simulink subsystem "StudentTemplate_M2"  (R2025a)
settings: Solver=VariableStepAuto  StartTime=0.0  StopTime=10.0  RelTol=1e-3
libraries: simulink x5, eeGeneralControl x3, slpidlib x2
settings Model: Creator=JesseJabezArendse  LastModifiedBy=MTMTAD006

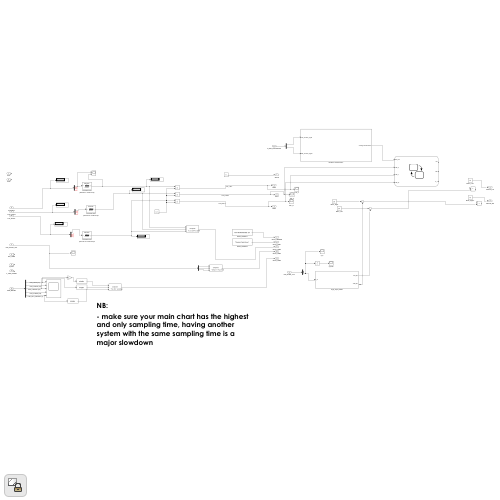
[thumbnail: Simulink's stored preview of the top-level diagram]
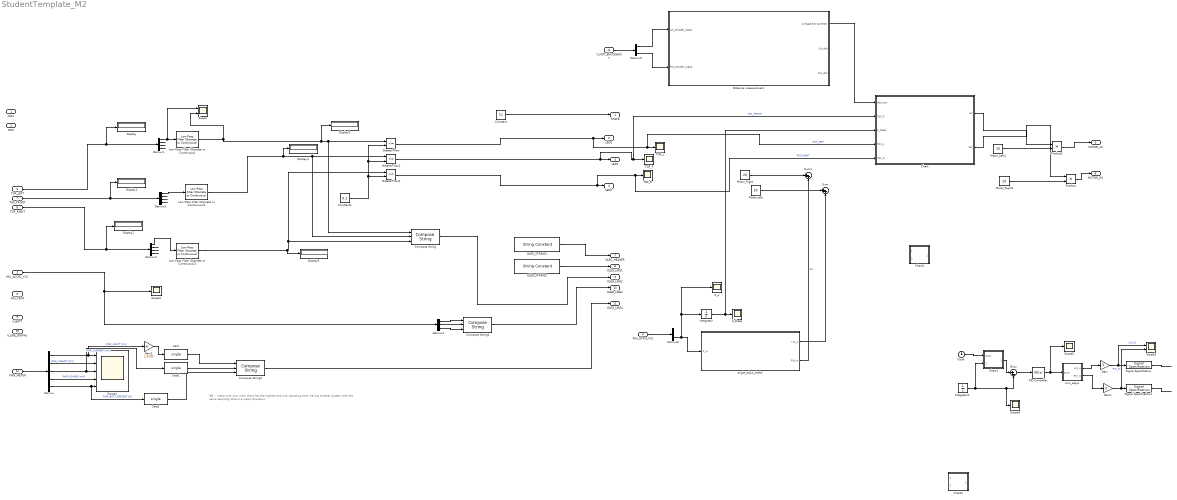
== system StudentTemplate_M2 ==
  note: NB:
      |
      | - make sure your main chart has the highest and only sampling time, having another system with the same sampling time is a major slowdown
  SW1 : Inport
  SW2 : Inport  Port=2
  IMU_ACCEL_XYZ : Inport  Port=3
  IMU_GYRO_XYZ : Inport  Port=4
  IMU_TEMP : Inport  Port=5
  TOF_LEFT : Inport  Port=6
  TOF_FRONT : Inport  Port=7
  TOF_RIGHT : Inport  Port=8
  V_BATT : Inport  Port=9
  V_LINE_DOWNs : Inport  Port=10
  V_MOT_ENCODERSs : Inport  Port=11
  PWR_METER : Inport  Port=12
  Cast : DataTypeConversion  OutDataTypeStr=single  SaturateOnIntegerOverflow=off  RndMeth=Floor
  Cast1 : DataTypeConversion  OutDataTypeStr=single  SaturateOnIntegerOverflow=off  RndMeth=Floor
  Cast2 : DataTypeConversion  OutDataTypeStr=single  SaturateOnIntegerOverflow=off  RndMeth=Floor
  Chart : Stateflow chart  TreatAsAtomicUnit=on
      settings: PortSchema="{\"entries\":[{\"content\":{\"sides\":[{\"content\":{\"connectorIds\":[\"In3\",\"In4\",\"In5\",\"In1\",\"In2\"]},\"type\":\"ConnectorPlacement.EquallySpacedRectSide\",\"uuid\":\"48a59af2-7c84-427a-8e2f-b10f2a044ed3\"},{\"content\":{\"connectorIds\":[\"Out1\",\"Out2\"],\"side\":\"RIGHT\"},\"type\":\"ConnectorPlacement.EquallySpacedRectSide\",\"uuid\":\"ddb5ed95-9874-42e8-8fee-75458ccb7c53\"},{\"content\":{\"side\":\"TOP\"},\"type\":\"ConnectorPlacement.EquallySpacedRectSide\",\"uuid\":\"d57417fe-864c-49b1-b704-1964fc5ecc42\"}]},\"type\":\"ConnectorPlacement.EquallySpacedConnector\",\"uuid\":\"f24c4a6d-faf6-462a-ab68-e289d44b6927\"}],\"packageUris\":[\"http://schema.mathworks.com/mf0/Connector/R2020b\"],\"version\":\"1.0\"}"
  Chart1 : Stateflow chart  TreatAsAtomicUnit=on
  Chart2 : Stateflow chart  TreatAsAtomicUnit=on
  Chart3 : Stateflow chart  TreatAsAtomicUnit=on
  Clock : Clock
  Compose String : ComposeString  Format="\"L%1.2f F%1.2f R%1.2f\""
  Compose String1 : ComposeString  Format="\"X%2.1f  Y%2.1f  Z%2.1f\""
  Compose String2 : ComposeString  Format="\"%1.2fV  %3.0fmA  %2.0f%%\""
  Constant : Constant  Value=11
  Constant1 : Constant  Value=0.1  SampleTime=-1
  "DIstance measurement " : Subsystem
  Demux : Demux  Outputs=5
  Demux1 : Demux
  Demux2 : Demux
  Demux3 : Demux
  Demux4 : Demux  Outputs=3
  Demux5 : Demux  Outputs=2
  Demux6 : Demux  Outputs=3
  Display{,1..5} (6 alike) : Display
  Error : Sum  Inputs=|+-
  Gain : Gain  Gain=5
  Gain1 : Gain  Gain=5
  Gain2 : Gain  Gain=1/1000
  GreaterThan : RelationalOperator  Operator=<=  OutDataTypeStr=boolean  RndMeth=Simplest  InputSameDT=off
  GreaterThan1 : RelationalOperator  Operator=<=  OutDataTypeStr=boolean  RndMeth=Simplest  InputSameDT=off
  GreaterThan2 : RelationalOperator  Operator=<=  OutDataTypeStr=boolean  RndMeth=Simplest  InputSameDT=off
  Integrator : Integrator
  Integrator1 : Integrator
  Low-Pass Filter (Discrete or Continuous) : eeGeneralControl/Low-Pass Filter (Discrete or Continuous)  K=1  T=0.1  B=inf  A=-inf  init_option=Inherited from block input  x0=0  Ts=-1
  Low-Pass Filter (Discrete or Continuous)1 : eeGeneralControl/Low-Pass Filter (Discrete or Continuous)  K=1  T=0.1  B=inf  A=-inf  init_option=Inherited from block input  x0=0  Ts=-1
  Low-Pass Filter (Discrete or Continuous)2 : eeGeneralControl/Low-Pass Filter (Discrete or Continuous)  K=1  T=0.1  B=inf  A=-inf  init_option=Inherited from block input  x0=0  Ts=-1
  Motor_Left : Constant  Value=20
  Motor_Left1 : Constant  Value=20
  Motor_Right : Constant  Value=20
  Motor_Right1 : Constant  Value=20
  OLED_STRING1 : StringConstant  String="\"UCT MICROMOUSE '25\""
  OLED_STRING2 : StringConstant  String="\"Simulink Data Demo\""
  PID Controller : slpidlib/PID Controller  Controller=PD  Form=Parallel  TimeDomain=Continuous-time  UseExternalTs=off  SampleTime=-1  IntegratorMethod=Forward Euler  FilterMethod=Forward Euler  ControllerParametersSource=internal  P=50  I=1  UseKiTs=off  D=1  UseExternalDerivativeSource=off  N=100  UseFilter=on  TunerSelectOption=Transfer Function Based (PID Tuner App)  InitialConditionSource=internal  InitialConditionForIntegrator=0  InitialConditionForFilter=0  DifferentiatorICPrevScaledInput=0  ExternalReset=none  TrackingMode=off  Kt=1  LimitOutput=off  SatLimitsSource=internal  UpperSaturationLimit=inf  LowerSaturationLimit=-inf  LinearizeAsGain=on  AntiWindupMode=none  Kb=1  LimitIntegrator=off  UpperIntegratorSaturationLimit=inf  LowerIntegratorSaturationLimit=-inf  POutMin=[]  POutMax=[]  IOutMin=[]  IOutMax=[]  DOutMin=[]  DOutMax=[]  NOutMin=[]  NOutMax=[]  SumOutMin=[]  SumOutMax=[]  SaturationOutMin=[]  SaturationOutMax=[]  PParamMin=[]  PParamMax=[]  IParamMin=[]  IParamMax=[]  DParamMin=[]  DParamMax=[]  NParamMin=[]  NParamMax=[]  KbParamMin=[]  KbParamMax=[]  KtParamMin=[]  KtParamMax=[]  KbOutMin=[]  KbOutMax=[]  KtOutMin=[]  KtOutMax=[]  IntegratorOutMin=[]  IntegratorOutMax=[]  FilterOutMin=[]  FilterOutMax=[]  SumI1OutMin=[]  SumI1OutMax=[]  SumI2OutMin=[]  SumI2OutMax=[]  SumI3OutMin=[]  SumI3OutMax=[]  SumI4OutMin=[]  SumI4OutMax=[]  SumDOutMin=[]  SumDOutMax=[]  DifferentiatorOutMin=[]  DifferentiatorOutMax=[]  FilterDiffOutCoefMin=[]  FilterDiffOutCoefMax=[]  ReciprocalOutMin=[]  ReciprocalOutMax=[]  SumDenOutMin=[]  SumDenOutMax=[]  SumNumOutMin=[]  SumNumOutMax=[]  DivideOutMin=[]  DivideOutMax=[]  UdiffTsProdOutMin=[]  UdiffTsProdOutMax=[]  NTsProdOutMin=[]  NTsProdOutMax=[]  UintegralTsProdOutMin=[]  UintegralTsProdOutMax=[]  UngainTsProdOutMin=[]  UngainTsProdOutMax=[]  ClampingZeroOutDataTypeStr=Inherit: Inherit via back propagation  ClampingZeroOutMin=[]  ClampingZeroOutMax=[]  FilterDenConstantOutDataTypeStr=Inherit: Inherit via back propagation  FilterDenConstantOutMin=[]  FilterDenConstantOutMax=[]  PCopyOutDataTypeStr=Inherit: Inherit via back propagation  PCopyOutMin=[]  PCopyOutMax=[]  NCopyOutDataTypeStr=Inherit: Inherit via back propagation  NCopyOutMin=[]  NCopyOutMax=[]  IntegratorContinuousStateAttributes=''  IntegratorStateMustResolveToSignalObject=off  IntegratorRTWStateStorageClass=Auto  FilterContinuousStateAttributes=''  FilterStateMustResolveToSignalObject=off  FilterRTWStateStorageClass=Auto  ParallelPVariant=InternalParameters  IdealPVariant=Disabled  IVariant=Disabled  DVariant=InternalParameters  IntegratorVariant=Disabled  SatVariant=Disabled  AWVariant=Disabled  PCopyVariant=Disabled  TRVariant=Disabled  FdbkBlocksVariant=Forward  IdealPFdbkVariant=Disabled  SatFdbkVariant=Disabled  DerivativeFilterVariant=ContFilter  NVariant=InternalParameters  NCopyVariant=Disabled  FilterICVariant=InternalICsFilter  IntegratorICVariant=Disabled  ExternalResetVariant=Disabled  TRSumVariant=Passthrough  SumFdbkVariant=Disabled  SumVariant=Sum_PD  TsampFilterVariant=InternalTs  TsampNgainVariant=Passthrough  TsampIntegralVariant=Disabled_SignalSpec  ExternalSaturationOutDataTypeStr=Inherit: Same as second input  DerivativeSourceVariant=ErrorSignal  PreIntVariant=InternalPreInt
  Product : Product
  Product1 : Product
  Scope : Scope  NumInputPorts=2
      settings: ActiveDisplayYMinimum=0.22759  ActiveDisplayYMaximum=0.52326
  Scope1 : Scope  NumInputPorts=5
      settings: ActiveDisplayYMinimum=-437.5  ActiveDisplayYMaximum=3937.5  DataLoggingVariableName=ScopeData2
  Scope2 : Scope
  Scope3 : Scope  NumInputPorts=2
      settings: ActiveDisplayYMinimum=-440.40684872460486  ActiveDisplayYMaximum=398.93122569343797  DataLoggingVariableName=ScopeData11
  Scope4 : Scope
      settings: ActiveDisplayYMinimum=-2.1976138852237335  ActiveDisplayYMaximum=0.12970641062525379  DataLoggingVariableName=ScopeData14
  Scope5 : Scope
      settings: ActiveDisplayYMinimum=-4.4488284675734473  ActiveDisplayYMaximum=3.9249085751009725  DataLoggingVariableName=ScopeData16
  Signal Specification : SignalSpecification  Dimensions=1
  Signal Specification1 : SignalSpecification  Dimensions=1
  Sum : Sum  Inputs=|++
  Sum1 : Sum  Inputs=|++
  TOF_F : Scope
      settings: ActiveDisplayYMinimum=-0.1769980412947128  ActiveDisplayYMaximum=0.90279895686963285  DataLoggingVariableName=ScopeData4
  TOF_L : Scope
      settings: ActiveDisplayYMinimum=-0.062899688908756052  ActiveDisplayYMaximum=0.13734742485444948  DataLoggingVariableName=ScopeData3
  TOF_R : Scope
      settings: ActiveDisplayYMinimum=0.84085955530656642  ActiveDisplayYMaximum=1.1222796398378163  DataLoggingVariableName=ScopeData5
  Z_theta : Scope
      settings: ActiveDisplayYMinimum=-2.70161604115423  ActiveDisplayYMaximum=4.8892356554264911  DataLoggingVariableName=ScopeData7
  Z_w : Scope
      settings: ActiveDisplayYMinimum=0.15654767663707053  ActiveDisplayYMaximum=0.20860795869615065  DataLoggingVariableName=ScopeData6
  angle_adjus_draft2 : Subsystem
  turn_adjus : Stateflow chart  TreatAsAtomicUnit=on
  STATE : Outport
  LED0 : Outport  Port=2
  LED1 : Outport  Port=3
  LED2 : Outport  Port=4
  MOTOR_LS : Outport  Port=5
  MOTOR_RS : Outport  Port=6
  OLED_HEADER : Outport  Port=7
  OLED_LINE1 : Outport  Port=8
  OLED_LINE2 : Outport  Port=9
  OLED_LINE3 : Outport  Port=10
  OLED_LINE4 : Outport  Port=11
  wires:
  TOF_FRONT/1 -> Demux3/1, Display1/1
  OLED_STRING2/1 -> OLED_LINE1/1
  Demux2/1 -> Low-Pass Filter (Discrete or Continuous)2/1
  Demux2/3 -> ?
  Demux2/2 -> ?
  Demux2/4 -> ?
  Compose String1/1 -> OLED_LINE3/1
  Low-Pass Filter (Discrete or Continuous)1/1 -> Compose String/2, GreaterThan1/1, Display4/1
  GreaterThan1/1 -> LED1/1, TOF_F/1, Chart/4(TOF_F)  "TOF_FRONT"
  Demux3/3 -> ?
  TOF_RIGHT/1 -> Demux2/1, Display2/1
  Demux3/4 -> ?
  Demux3/2 -> ?
  Demux1/2 -> ?
  Demux3/1 -> Low-Pass Filter (Discrete or Continuous)1/1
  OLED_STRING1/1 -> OLED_HEADER/1
  Demux1/1 -> Scope/1, Low-Pass Filter (Discrete or Continuous)/1
  Compose String/1 -> OLED_LINE2/1
  Constant1/1 -> GreaterThan2/2, GreaterThan1/2, GreaterThan/2
  Demux1/4 -> ?
  GreaterThan2/1 -> TOF_R/1, Chart/2(TOF_R), LED2/1  "TOF_RIGHT"
  TOF_LEFT/1 -> Demux1/1, Display/1
  GreaterThan/1 -> LED0/1, TOF_L/1, Chart/1(TOF_L)  "TOF_LEFT"
  Demux1/3 -> ?
  PWR_METER/1 -> Demux/1
  Demux/1 -> Scope1/1, Gain2/1  "PWR_VBATT [mV]"
  Demux/2 -> Scope1/2  "PWR_VSHUNT [mV]"
  Demux/3 -> Scope1/3, Cast1/1  "PWR_CURRENT [mA]"
  Demux/4 -> Scope1/4  "PWR_POWER [mW]"
  Demux/5 -> Scope1/5, Cast2/1  "PWR_BATT_PERCENT [%]"
  IMU_ACCEL_XYZ/1 -> Demux4/1, Scope2/1
  Demux4/1 -> Compose String1/1
  Demux4/2 -> Compose String1/2
  Demux4/3 -> Compose String1/3
  Compose String2/1 -> OLED_LINE4/1
  Gain2/1 -> Cast/1
  Cast/1 -> Compose String2/1
  Cast1/1 -> Compose String2/2
  Cast2/1 -> Compose String2/3
  Low-Pass Filter (Discrete or Continuous)2/1 -> Compose String/3, GreaterThan2/1, Display5/1
  Low-Pass Filter (Discrete or Continuous)/1 -> Scope/2, Compose String/1, GreaterThan/1, Display3/1
  Constant/1 -> STATE/1
  Motor_Right/1 -> Sum1/1
  V_MOT_ENCODERSs/1 -> Demux5/1
  Demux5/1 -> "DIstance measurement "/1(LW_encoder_signal)
  Demux5/2 -> "DIstance measurement "/2(RW_encoder_signal)
  IMU_GYRO_XYZ/1 -> Demux6/1
  Demux6/3 -> angle_adjus_draft2/1(Z_w), Integrator/1, Z_w/1
  Motor_Left/1 -> Sum/1
  angle_adjus_draft2/1(LW_w) -> Sum/2
  angle_adjus_draft2/2(RW_w) -> Sum1/2  "RW"
  Motor_Left1/1 -> Product1/2
  Motor_Right1/1 -> Product/2
  "DIstance measurement "/1("Average dist tarvelled ") -> Chart/3(dist_trav)
  Product1/1 -> MOTOR_LS/1
  Product/1 -> MOTOR_RS/1
  Integrator/1 -> Z_theta/1, Chart/5(Z_theta)
  Chart/2(RW) -> Product/1
  Chart/1(LW) -> Product1/1
  Clock/1 -> Chart1/1(clock)
  Error/1 -> PID Controller/1
  Signal Specification/1 -> ?
  turn_adjus/1(LW_w) -> Gain/1
  turn_adjus/2(RW_w) -> Gain1/1
  Gain1/1 -> Signal Specification1/1, Scope3/2  "RW_W"
  Integrator1/1 -> Error/2, Scope4/1, Chart1/2(Z_theta)
  Chart1/1(offset) -> Error/1
  Signal Specification1/1 -> ?
  PID Controller/1 -> turn_adjus/1(error), Scope5/1
  Gain/1 -> Signal Specification/1, Scope3/1  "LW_W"

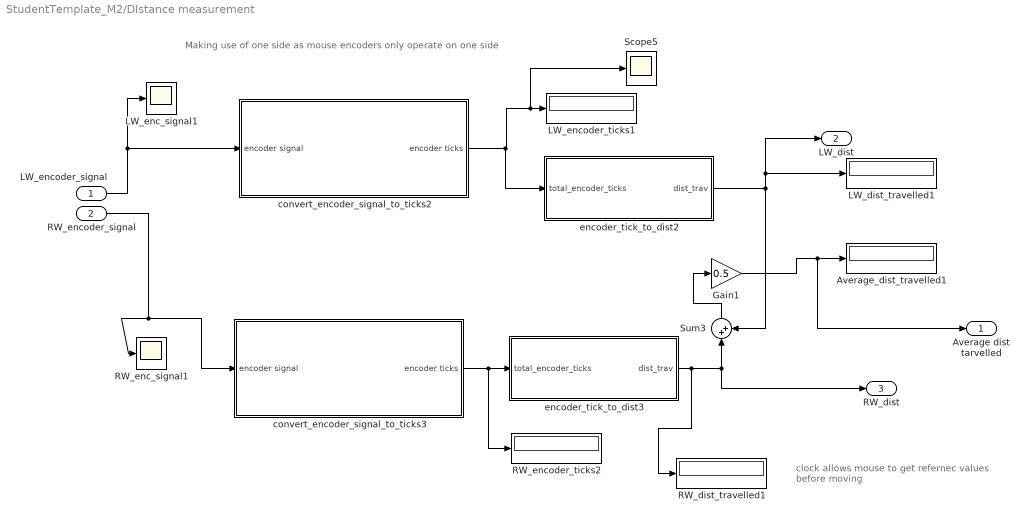
== system StudentTemplate_M2/DIstance measurement  ==
  note: Making use of one side as mouse encoders only operate on one side
  note: clock allows mouse to get refernec values
      | before moving
  LW_encoder_signal : Inport
  RW_encoder_signal : Inport  Port=2
  Average_dist_travelled1 : Display
  Gain1 : Gain  Gain=0.5
  LW_dist_travelled1 : Display
  LW_enc_signal1 : Scope
      settings: ActiveDisplayYMinimum=-1.5423087408726712  ActiveDisplayYMaximum=1.7466656009006407  DataLoggingVariableName=ScopeData13
  LW_encoder_ticks1 : Display
  RW_dist_travelled1 : Display
  RW_enc_signal1 : Scope
      settings: ActiveDisplayYMinimum=-1.944570956862778  ActiveDisplayYMaximum=2.0482644886882531  DataLoggingVariableName=ScopeData15
  RW_encoder_ticks2 : Display
  Scope5 : Scope
      settings: ActiveDisplayYMinimum=68.495784543089613  ActiveDisplayYMaximum=92.847652845801534  DataLoggingVariableName=ScopeData18
  Sum3 : Sum  Inputs=|++
  convert_encoder_signal_to_ticks2 : Subsystem
  convert_encoder_signal_to_ticks3 : Subsystem
  encoder_tick_to_dist2 : Subsystem
  encoder_tick_to_dist3 : Subsystem
  "Average dist tarvelled " : Outport
  LW_dist : Outport  Port=2
  RW_dist : Outport  Port=3
  wires:
  LW_encoder_signal/1 -> convert_encoder_signal_to_ticks2/1(encoder signal), LW_enc_signal1/1
  encoder_tick_to_dist3/1(dist_trav) -> RW_dist_travelled1/1, RW_dist/1, Sum3/1
  convert_encoder_signal_to_ticks3/1(encoder ticks) -> RW_encoder_ticks2/1, encoder_tick_to_dist3/1(total_encoder_ticks)
  Sum3/1 -> Gain1/1
  convert_encoder_signal_to_ticks2/1(encoder ticks) -> encoder_tick_to_dist2/1(total_encoder_ticks), Scope5/1, LW_encoder_ticks1/1
  Gain1/1 -> Average_dist_travelled1/1, "Average dist tarvelled "/1
  RW_encoder_signal/1 -> RW_enc_signal1/1, convert_encoder_signal_to_ticks3/1(encoder signal)
  encoder_tick_to_dist2/1(dist_trav) -> Sum3/2, LW_dist_travelled1/1, LW_dist/1

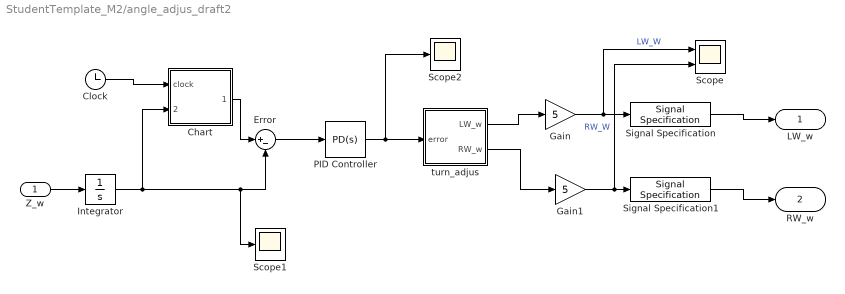
== system StudentTemplate_M2/angle_adjus_draft2 ==
  Z_w : Inport
  Chart : Stateflow chart  TreatAsAtomicUnit=on
  Clock : Clock
  Error : Sum  Inputs=|+-
  Gain : Gain  Gain=5
  Gain1 : Gain  Gain=5
  Integrator : Integrator
  PID Controller : slpidlib/PID Controller  Controller=PD  Form=Parallel  TimeDomain=Continuous-time  UseExternalTs=off  SampleTime=-1  IntegratorMethod=Forward Euler  FilterMethod=Forward Euler  ControllerParametersSource=internal  P=50  I=1  UseKiTs=off  D=1  UseExternalDerivativeSource=off  N=100  UseFilter=on  TunerSelectOption=Transfer Function Based (PID Tuner App)  InitialConditionSource=internal  InitialConditionForIntegrator=0  InitialConditionForFilter=0  DifferentiatorICPrevScaledInput=0  ExternalReset=none  TrackingMode=off  Kt=1  LimitOutput=off  SatLimitsSource=internal  UpperSaturationLimit=inf  LowerSaturationLimit=-inf  LinearizeAsGain=on  AntiWindupMode=none  Kb=1  LimitIntegrator=off  UpperIntegratorSaturationLimit=inf  LowerIntegratorSaturationLimit=-inf  POutMin=[]  POutMax=[]  IOutMin=[]  IOutMax=[]  DOutMin=[]  DOutMax=[]  NOutMin=[]  NOutMax=[]  SumOutMin=[]  SumOutMax=[]  SaturationOutMin=[]  SaturationOutMax=[]  PParamMin=[]  PParamMax=[]  IParamMin=[]  IParamMax=[]  DParamMin=[]  DParamMax=[]  NParamMin=[]  NParamMax=[]  KbParamMin=[]  KbParamMax=[]  KtParamMin=[]  KtParamMax=[]  KbOutMin=[]  KbOutMax=[]  KtOutMin=[]  KtOutMax=[]  IntegratorOutMin=[]  IntegratorOutMax=[]  FilterOutMin=[]  FilterOutMax=[]  SumI1OutMin=[]  SumI1OutMax=[]  SumI2OutMin=[]  SumI2OutMax=[]  SumI3OutMin=[]  SumI3OutMax=[]  SumI4OutMin=[]  SumI4OutMax=[]  SumDOutMin=[]  SumDOutMax=[]  DifferentiatorOutMin=[]  DifferentiatorOutMax=[]  FilterDiffOutCoefMin=[]  FilterDiffOutCoefMax=[]  ReciprocalOutMin=[]  ReciprocalOutMax=[]  SumDenOutMin=[]  SumDenOutMax=[]  SumNumOutMin=[]  SumNumOutMax=[]  DivideOutMin=[]  DivideOutMax=[]  UdiffTsProdOutMin=[]  UdiffTsProdOutMax=[]  NTsProdOutMin=[]  NTsProdOutMax=[]  UintegralTsProdOutMin=[]  UintegralTsProdOutMax=[]  UngainTsProdOutMin=[]  UngainTsProdOutMax=[]  ClampingZeroOutDataTypeStr=Inherit: Inherit via back propagation  ClampingZeroOutMin=[]  ClampingZeroOutMax=[]  FilterDenConstantOutDataTypeStr=Inherit: Inherit via back propagation  FilterDenConstantOutMin=[]  FilterDenConstantOutMax=[]  PCopyOutDataTypeStr=Inherit: Inherit via back propagation  PCopyOutMin=[]  PCopyOutMax=[]  NCopyOutDataTypeStr=Inherit: Inherit via back propagation  NCopyOutMin=[]  NCopyOutMax=[]  IntegratorContinuousStateAttributes=''  IntegratorStateMustResolveToSignalObject=off  IntegratorRTWStateStorageClass=Auto  FilterContinuousStateAttributes=''  FilterStateMustResolveToSignalObject=off  FilterRTWStateStorageClass=Auto  ParallelPVariant=InternalParameters  IdealPVariant=Disabled  IVariant=Disabled  DVariant=InternalParameters  IntegratorVariant=Disabled  SatVariant=Disabled  AWVariant=Disabled  PCopyVariant=Disabled  TRVariant=Disabled  FdbkBlocksVariant=Forward  IdealPFdbkVariant=Disabled  SatFdbkVariant=Disabled  DerivativeFilterVariant=ContFilter  NVariant=InternalParameters  NCopyVariant=Disabled  FilterICVariant=InternalICsFilter  IntegratorICVariant=Disabled  ExternalResetVariant=Disabled  TRSumVariant=Passthrough  SumFdbkVariant=Disabled  SumVariant=Sum_PD  TsampFilterVariant=InternalTs  TsampNgainVariant=Passthrough  TsampIntegralVariant=Disabled_SignalSpec  ExternalSaturationOutDataTypeStr=Inherit: Same as second input  DerivativeSourceVariant=ErrorSignal  PreIntVariant=InternalPreInt
  Scope : Scope  NumInputPorts=2
      settings: ActiveDisplayYMinimum=-440.40684872460486  ActiveDisplayYMaximum=398.93122569343797  DataLoggingVariableName=ScopeData8
  Scope1 : Scope
      settings: ActiveDisplayYMinimum=-2.1976138852237335  ActiveDisplayYMaximum=0.12970641062525379  DataLoggingVariableName=ScopeData12
  Scope2 : Scope
      settings: ActiveDisplayYMinimum=-4.4488284675734473  ActiveDisplayYMaximum=3.9249085751009725  DataLoggingVariableName=ScopeData10
  Signal Specification : SignalSpecification  Dimensions=1
  Signal Specification1 : SignalSpecification  Dimensions=1
  turn_adjus : Stateflow chart  TreatAsAtomicUnit=on
  LW_w : Outport
  RW_w : Outport  Port=2
  wires:
  Clock/1 -> Chart/1(clock)
  Gain1/1 -> Signal Specification1/1, Scope/2  "RW_W"
  Gain/1 -> Signal Specification/1, Scope/1  "LW_W"
  Chart/1(offset) -> Error/1
  Z_w/1 -> Integrator/1
  Signal Specification1/1 -> RW_w/1
  Signal Specification/1 -> LW_w/1
  turn_adjus/2(RW_w) -> Gain1/1
  turn_adjus/1(LW_w) -> Gain/1
  PID Controller/1 -> turn_adjus/1(error), Scope2/1
  Error/1 -> PID Controller/1
  Integrator/1 -> Error/2, Scope1/1, Chart/2(Z_theta)

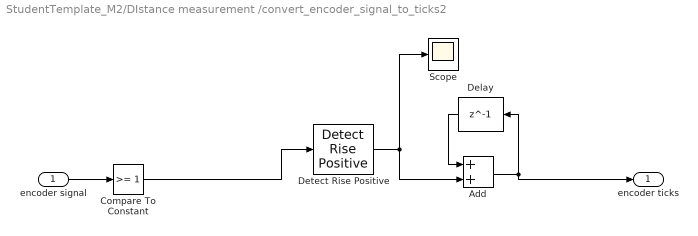
== system StudentTemplate_M2/DIstance measurement /convert_encoder_signal_to_ticks2 ==
  encoder signal : Inport
  Add : Sum
  Compare To Constant : simulink/Logic and Bit Operations/Compare To Constant  relop=>=  const=1  OutDataTypeStr=boolean
  Delay : Delay  DelayLength=1  InitialCondition=0
  Detect Rise Positive : simulink/Logic and Bit Operations/Detect Rise Positive  vinit=0  OutDataTypeStr=uint8
  Scope : Scope
      settings: ActiveDisplayYMinimum=-0.30381603839463822  ActiveDisplayYMaximum=1.4550594899256748  DataLoggingVariableName=ScopeData9
  encoder ticks : Outport
  wires:
  Add/1 -> encoder ticks/1, Delay/1
  Compare To Constant/1 -> Detect Rise Positive/1
  Detect Rise Positive/1 -> Add/2, Scope/1
  encoder signal/1 -> Compare To Constant/1
  Delay/1 -> Add/1

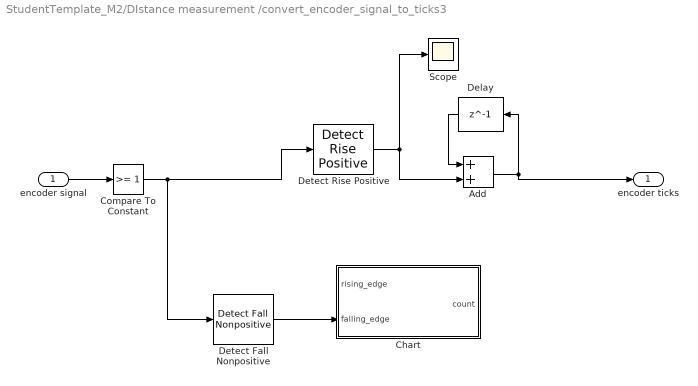
== system StudentTemplate_M2/DIstance measurement /convert_encoder_signal_to_ticks3 ==
  encoder signal : Inport
  Add : Sum
  Chart : Stateflow chart  TreatAsAtomicUnit=on
  Compare To Constant : simulink/Logic and Bit Operations/Compare To Constant  relop=>=  const=1  OutDataTypeStr=boolean
  Delay : Delay  DelayLength=1  InitialCondition=0
  Detect Fall Nonpositive : simulink/Logic and Bit Operations/Detect Fall Nonpositive  vinit=0  OutDataTypeStr=boolean
  Detect Rise Positive : simulink/Logic and Bit Operations/Detect Rise Positive  vinit=0  OutDataTypeStr=uint8
  Scope : Scope
      settings: ActiveDisplayYMinimum=-0.30381603839463822  ActiveDisplayYMaximum=1.4550594899256748  DataLoggingVariableName=ScopeData9
  encoder ticks : Outport
  wires:
  Add/1 -> encoder ticks/1, Delay/1
  Compare To Constant/1 -> Detect Fall Nonpositive/1, Detect Rise Positive/1
  Detect Rise Positive/1 -> Add/2, Scope/1
  encoder signal/1 -> Compare To Constant/1
  Delay/1 -> Add/1
  Detect Fall Nonpositive/1 -> Chart/2(falling_edge)

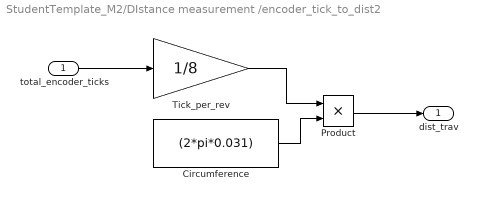
== system StudentTemplate_M2/DIstance measurement /encoder_tick_to_dist2 ==
  total_encoder_ticks : Inport
  Circumference : Constant  Value=(2*pi*0.031)
  Product : Product
  Tick_per_rev : Gain  Gain=1/8
  dist_trav : Outport
  wires:
  Product/1 -> dist_trav/1
  Tick_per_rev/1 -> Product/1
  Circumference/1 -> Product/2
  total_encoder_ticks/1 -> Tick_per_rev/1

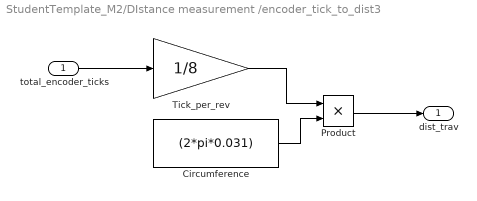
== system StudentTemplate_M2/DIstance measurement /encoder_tick_to_dist3 ==
  total_encoder_ticks : Inport
  Circumference : Constant  Value=(2*pi*0.031)
  Product : Product
  Tick_per_rev : Gain  Gain=1/8
  dist_trav : Outport
  wires:
  Product/1 -> dist_trav/1
  Tick_per_rev/1 -> Product/1
  Circumference/1 -> Product/2
  total_encoder_ticks/1 -> Tick_per_rev/1

== stateflow chart StudentTemplate_M2/Chart1 ==
  state Start
    during:
    offset= 0;
  state Set_Offset
    during:
    offset = Z_theta;
  (default) -> Start
  Start -> Set_Offset : [clock <0.1]
  Set_Offset -> Set_Offset : [clock > 0.1]
  data: clock input; offset output; Z_theta input

== stateflow chart StudentTemplate_M2/turn_adjus ==
  state deafult
    during:
    LW_w = 0;
    RW_w = 0;
  state turnLeft
    during:
    LW_w=-error;
    RW_w = error;
  state turnRight
    during:
    RW_w = error;
    LW_w = -error;
  (default) -> deafult
  deafult -> turnLeft [order 2] : [error>0 ]
  deafult -> turnRight [order 1] : [error<0 ]
  data: error input; LW_w output; RW_w output

== stateflow chart StudentTemplate_M2/Chart2 ==
  state Default
    entry:
    sum = TOF_L + TOF_R;
    during:
    reference = sum/2;
  (default) -> Default
  data: TOF_L input; TOF_R input; sum local; reference output

== stateflow chart StudentTemplate_M2/DIstance measurement /convert_encoder_signal_to_ticks3/Chart ==
  state default
    during:
    count =0;
  state encoder_pulse_start
    during:
  state encoder_pulse_end
    during:
    count = 1;
  (default) -> default
  default -> encoder_pulse_start : [rising_edge == 1]
  encoder_pulse_start -> encoder_pulse_end : [falling_edge == 1]
  data: rising_edge input; count output; falling_edge input

== stateflow chart StudentTemplate_M2/Chart3 ==
  state Default
    entry:
    sum = TOF_L + TOF_R;
    during:
    reference = sum/2;
  (default) -> Default
  data: TOF_L input; TOF_R input; sum local; reference output

== stateflow chart StudentTemplate_M2/angle_adjus_draft2/turn_adjus ==
  state deafult
    during:
    LW_w = 0;
    RW_w = 0;
  state turnLeft
    during:
    LW_w=-error;
    RW_w = error;
  state turnRight
    during:
    RW_w = error;
    LW_w = -error;
  (default) -> deafult
  deafult -> turnLeft [order 2] : [error>0 ]
  deafult -> turnRight [order 1] : [error<0 ]
  data: error input; LW_w output; RW_w output

== stateflow chart StudentTemplate_M2/angle_adjus_draft2/Chart ==
  state Start
    during:
    offset= 0;
  state Set_Offset
    during:
    offset = Z_theta;
  (default) -> Start
  Start -> Set_Offset : [clock <0.1]
  Set_Offset -> Set_Offset : [clock > 0.1]
  data: clock input; offset output; Z_theta input

== stateflow chart StudentTemplate_M2/Chart ==
  settings: updateMethod=CONTINUOUS
  state INIT
    entry:
    LW = 1;
    RW = 1;
  state Rotate
    entry:
    LW = 0;
    RW = 0;
    during:
    RW = 1;
    LW = -1;
  state trn_left_init
    entry:
    start_dist = dist_trav;
    LW = 0;
    RW = 0;
  state Postion_robot
    entry:
    end_dist = start_dist + 0.11;
    LW = 0.5;
    RW =0.5;
  state Rotate1
    entry:
    LW = 0;
    RW = 0;
    during:
    RW = -1;
    LW = 1;
  state trn_right_init1
    entry:
    start_dist = dist_trav;
    LW = 0;
    RW = 0;
  state Postion_robot1
    entry:
    end_dist = start_dist + 0.11;
    LW = 0.5;
    RW =0.5;
  (default) -> INIT
  trn_left_init -> Postion_robot [order 2] : after(2,sec) [TOF_L == 0]
  Postion_robot -> Rotate [order 2] : [dist_trav >= end_dist]
  INIT -> trn_left_init [order 1] : [TOF_R == 1 && TOF_L == 0]
  INIT -> trn_right_init1 [order 2] : [TOF_R == 0 && TOF_L == 1]
  (junction 20) -> INIT
  trn_left_init -> (junction 21) [order 1] : [TOF_L ==1]
  Postion_robot -> (junction 53) [order 1] : [TOF_F == 1]
  Rotate -> (junction 58) : [Z_theta >= pi/2]
  (junction 58) -> (junction 53)
  (junction 53) -> (junction 21)
  (junction 21) -> (junction 20)
  trn_right_init1 -> (junction 20) [order 2] : [TOF_R == 1]
  Rotate1 -> (junction 53) : [Z_theta >= pi/2]
  Postion_robot1 -> Rotate1 : [dist_trav >= end_dist]
  trn_right_init1 -> Postion_robot1 [order 1] : [TOF_R == 0]
  data: TOF_L input; TOF_R input; LW output; RW output; dist_trav input; start_dist local; TOF_F input; end_dist local; Z_theta input
